simulink model "mpc_v0_1"  (R2020b)
settings: Solver=ode4  StartTime=0.0  StopTime=t_sim  FixedStep=T  RelTol=1e-3
values from neighbouring files (symbols this model uses):
  ref = [18; 9; 0; 0]    [main_01.m]
  T = 0.01    [main_01.m]
  x0 = [1; 1; 0; 0]    [main_01.m]
undefined symbols (not defined in the file or in its folder): map, mpc, mpc_param
settings Model: SimulationMode=accelerator  Creator=vince  LastModifiedBy=vince
settings DataIOCC: ReturnWorkspaceOutputs=off

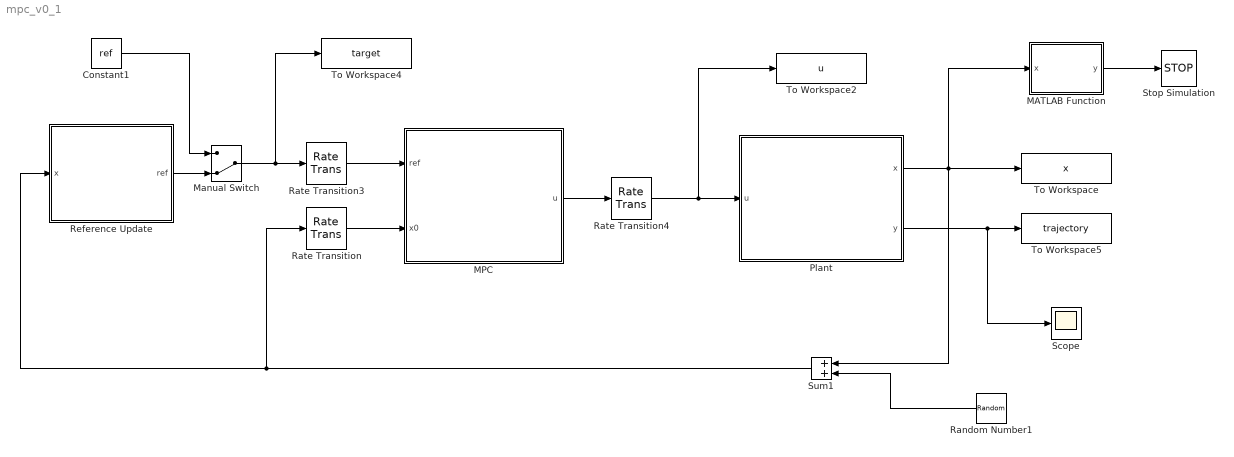
== system mpc_v0_1 ==
  Constant1 : Constant  Value=ref  SampleTime=-1
  MATLAB Function : MATLAB Function  TreatAsAtomicUnit=on
  MPC : Subsystem
  Manual Switch : ManualSwitch  CurrentSetting=0
  Plant : Subsystem
  Random Number1 : RandomNumber  Variance=0
  Rate Transition : RateTransition  OutPortSampleTime=mpc.Ts
  Rate Transition3 : RateTransition  OutPortSampleTime=mpc.Ts
  Rate Transition4 : RateTransition  OutPortSampleTime=T
  Reference Update : Subsystem
  Scope : Scope
  Stop Simulation : Stop
  Sum1 : Sum
  To Workspace : ToWorkspace  VariableName=x  SaveFormat=Timeseries  SampleTime=-1
  To Workspace2 : ToWorkspace  VariableName=u  SaveFormat=Timeseries  SampleTime=-1
  To Workspace4 : ToWorkspace  VariableName=target  SaveFormat=Timeseries  SampleTime=-1
  To Workspace5 : ToWorkspace  VariableName=trajectory  SaveFormat=Timeseries  SampleTime=-1
  wires:
  Rate Transition4/1 -> To Workspace2/1, Plant/1(u)
  MPC/1(u) -> Rate Transition4/1
  Rate Transition3/1 -> MPC/1(ref)
  Rate Transition/1 -> MPC/2(x0)
  Plant/2(y) -> Scope/1, To Workspace5/1
  Reference Update/1(ref) -> Manual Switch/2
  Constant1/1 -> Manual Switch/1
  Manual Switch/1 -> To Workspace4/1, Rate Transition3/1
  MATLAB Function/1(y) -> Stop Simulation/1
  Plant/1(x) -> Sum1/1, MATLAB Function/1(x), To Workspace/1
  Random Number1/1 -> Sum1/2
  Sum1/1 -> Rate Transition/1, Reference Update/1(x)

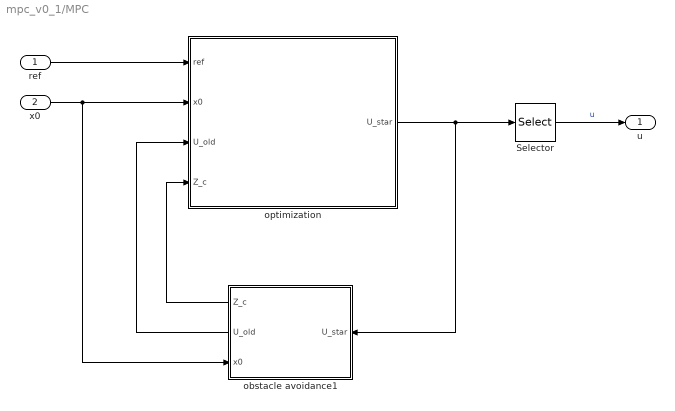
== system mpc_v0_1/MPC ==
  ref : Inport
  x0 : Inport  Port=2
  Selector : Selector  InputPortWidth=mpc.q*mpc.Nc  IndexOptions=Index vector (dialog)  Indices=1:mpc.q  OutputSizes=1
  obstacle avoidance1 : Subsystem
      settings: PortSchema="{\"entries\":[{\"content\":{\"sides\":[{\"content\":{\"connectorIds\":[\"Out1\",\"Out2\",\"In1\"]},\"type\":\"ConnectorPlacement.EquallySpacedRectSide\",\"uuid\":\"6e6bb291-76b9-457f-8d04-015292ad1700\"},{\"content\":{\"connectorIds\":[\"In2\"],\"side\":\"RIGHT\"},\"type\":\"ConnectorPlacement.EquallySpacedRectSide\",\"uuid\":\"1fce423a-e385-4f15-9cbd-eabef89b0aaa\"},{\"content\":{\"connectorIds\":[],\"side\":\"TOP\"},\"type\":\"ConnectorPlacement.EquallySpacedRectSide\",\"uuid\":\"fdf64715-349b-4f23-8b41-9be7dc47d341\"},{\"content\":{\"connectorIds\":[],\"side\":\"HIDDEN\"},\"type\":\"ConnectorPlacement.EquallySpacedRectSide\",\"uuid\":\"ad220cca-5aec-45e2-9094-855ca00bdb40\"}]},\"type\":\"ConnectorPlacement.EquallySpacedConnector\",\"uuid\":\"3c5e2d21-75ff-4523-ba4d-4cc947bcae8c\"}],\"packageUris\":[\"http://schema.mathworks.com/mf0/Connector/R2020b\"],\"version\":\"1.0\"}"
  optimization : MATLAB Function  TreatAsAtomicUnit=on
  u : Outport
  wires:
  ref/1 -> optimization/1(ref)
  x0/1 -> obstacle avoidance1/1(x0), optimization/2(x0)
  Selector/1 -> u/1  "u"
  obstacle avoidance1/1(Z_c) -> optimization/4(Z_c)
  optimization/1(U_star) -> obstacle avoidance1/2(U_star), Selector/1
  obstacle avoidance1/2(U_old) -> optimization/3(U_old)

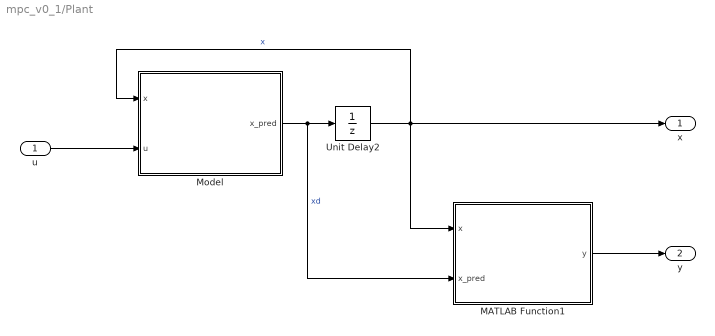
== system mpc_v0_1/Plant ==
  u : Inport
  MATLAB Function1 : MATLAB Function  TreatAsAtomicUnit=on
  Model : MATLAB Function  TreatAsAtomicUnit=on
  Unit Delay2 : UnitDelay  InitialCondition=x0  SampleTime=T  HasFrameUpgradeWarning=on
  x : Outport
  y : Outport  Port=2
  wires:
  u/1 -> Model/2(u)
  Unit Delay2/1 -> MATLAB Function1/1(x), Model/1(x), x/1  "x"
  MATLAB Function1/1(y) -> y/1
  Model/1(x_pred) -> MATLAB Function1/2(x_pred), Unit Delay2/1  "xd"

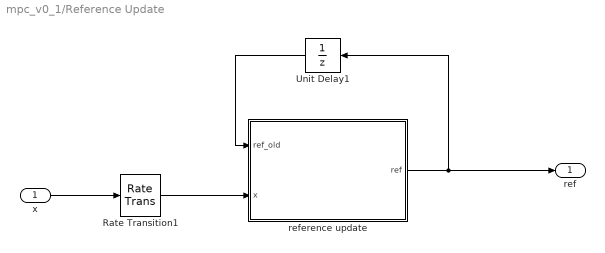
== system mpc_v0_1/Reference Update ==
  x : Inport
  Rate Transition1 : RateTransition  OutPortSampleTime=T
  Unit Delay1 : UnitDelay  InitialCondition=zeros(mpc_param.p,1)  SampleTime=T  HasFrameUpgradeWarning=on
  reference update : MATLAB Function  TreatAsAtomicUnit=on
  ref : Outport
  wires:
  Unit Delay1/1 -> reference update/1(ref_old)
  x/1 -> Rate Transition1/1
  reference update/1(ref) -> Unit Delay1/1, ref/1
  Rate Transition1/1 -> reference update/2(x)

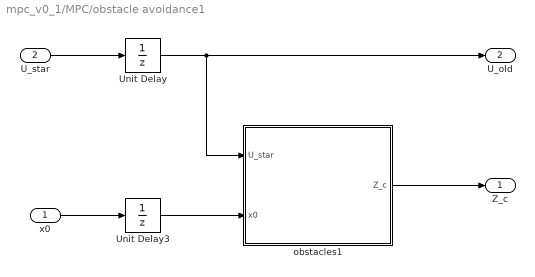
== system mpc_v0_1/MPC/obstacle avoidance1 ==
  x0 : Inport
  U_star : Inport  Port=2
  Unit Delay : UnitDelay  InitialCondition=zeros(mpc.q*mpc.Nc, 1)  SampleTime=mpc.Ts  HasFrameUpgradeWarning=on
  Unit Delay3 : UnitDelay  InitialCondition=x0  SampleTime=mpc.Ts  HasFrameUpgradeWarning=on
  obstacles1 : MATLAB Function  TreatAsAtomicUnit=on
  Z_c : Outport
  U_old : Outport  Port=2
  wires:
  obstacles1/1(Z_c) -> Z_c/1
  U_star/1 -> Unit Delay/1
  Unit Delay3/1 -> obstacles1/2(x0)
  x0/1 -> Unit Delay3/1
  Unit Delay/1 -> obstacles1/1(U_star), U_old/1

== matlab function mpc_v0_1/MPC/obstacle avoidance1/obstacles1 ==
  data: U_star input; x0 input; Z_c output; mpc parameter; map parameter
function Z_c = obstacles(U_star, x0, mpc, map)


%% Initialization
x_c = NaN*ones(mpc.Np,2);
y_c = NaN*ones(mpc.Np,2);
z_c = zeros(mpc.p*mpc.Np, 2);



%% Predicted output
X_p = mpc.A_bar*x0 + mpc.B_bar*U_star;
X = X_p(1:4:end);
Y = X_p(2:4:end);



%% Update constraints

for j = 1:mpc.Np
    %% X_c
    k = 1;
    
    for i = 1:length(map.Sx)
        if (abs(X(j)-map.Sx(i,1))>map.r_act)
            continue;
        end
        if (map.Sx(i,2)<=Y(j) && Y(j)<=map.Sx(i,3))
            x_c(j,k) = map.Sx(i,1);
            k = k+1;
        end
        if k>2
            break;
        end
    end
    

    if (isnan(x_c(j,1)) && isnan(x_c(j,2)))
        x_c(j,:) = [-Inf +Inf];
    elseif (isnan(x_c(j,2)) && X(j)>x_c(j,1))
        x_c(j,1) = x_c(j,1);
        x_c(j,2) = +Inf;
    elseif (isnan(x_c(j,2)) && X(j)<x_c(j,1))
        x_c(j,2) = x_c(j,1);
        x_c(j,1) = -Inf;
    end
    
    
    
    %% Y_c
    k = 1;

    for i=1:length(map.Sy)
        if (abs(Y(j)-map.Sy(i,1))>map.r_act)
            continue;
        end
        
        if (map.Sy(i,2)<=X(j) && X(j)<=map.Sy(i,3))
            y_c(j,k) = map.Sy(i,1);
            k = k+1;
        end
          
        if k>2
            break;
        end
    end
    
    
    if (isnan(y_c(j,1)) && isnan(y_c(j,2)))
        y_c(j,:) = [-Inf +Inf];
    elseif (isnan(y_c(j,2)) && Y(j)>y_c(j,1))
        y_c(j,1) = y_c(j,1);
        y_c(j,2) = +Inf;
    elseif (isnan(y_c(j,2)) && Y(j)<y_c(j,1))
        y_c(j,2) = y_c(j,1);
        y_c(j,1) = -Inf;
    end
    
    
    %% 
    z_c(2*j-1:2*j,:) = [x_c(j,1)+map.r_safe x_c(j,2)-map.r_safe; 
                        y_c(j,1)+map.r_safe y_c(j,2)-map.r_safe];


end


% X_min = x_c(1,1);
% X_max = x_c(1,2);
% Y_min = y_c(1,1);
% Y_max = y_c(1,2);

Z_c = z_c;

== matlab function mpc_v0_1/MPC/optimization ==
  data: ref input; U_star output; x0 input; U_old input; Z_c input; mpc parameter
function U_star   = mpc_optimization(ref, x0, U_old, Z_c, mpc)
%% Documentation
%{
    IN: ref, x, U_old
    OUT: U*
%}


%% Reference
REF = repmat(ref, mpc.Np, 1);



%% Constraints
X_min = mpc.X_c(:,1);
X_max = mpc.X_c(:,2);
% for i=1:mpc.Np
%     X_min((mpc.n*i)-3:(mpc.n*i)-2, 1) = Z_c((2*i)-1:2*i, 1);
%     X_max((mpc.n*i)-3:(mpc.n*i)-2, 1) = Z_c((2*i)-1:2*i, 2);
% end
U_min = mpc.U_c(:,1);
U_max = mpc.U_c(:,2);
dU_min = mpc.dU_c(:,1);
dU_max = mpc.dU_c(:,2);

A_ineq = [-mpc.B_bar; 
          mpc.B_bar;
          -eye(mpc.q*mpc.Nc); 
          eye(mpc.q*mpc.Nc); 
          -eye(mpc.q*mpc.Nc); 
          eye(mpc.q*mpc.Nc)];
b_ineq = [-X_min+mpc.A_bar*x0; 
          X_max-mpc.A_bar*x0;
          -U_min; 
          U_max;
          -dU_min-U_old; 
          dU_max+U_old];



%% Objective function
H = mpc.R_bar + mpc.D_bar'*mpc.Q_bar*mpc.D_bar;
H = (H+H')/2;
f = (mpc.C_bar*x0-REF)'*mpc.Q_bar*(mpc.D_bar);



%% Optimization: J(u(k)) = U(k)'*H*U(k) + f'*U(k)
coder.extrinsic('quadprog');
% options = optimoptions('quadprog', 'Algorithm', 'active-set', 'Display', 'iter');

U_star = zeros(mpc.q*mpc.Nc, 1);
U_star = quadprog(H, f, A_ineq, b_ineq, [], [], [], [], []);

== matlab function mpc_v0_1/Plant/Model ==
  data: x input; u input; x_pred output; T parameter
function x_pred = mpc_pred_disc(x, u, T)


A = [0 0 1 0; 0 0 0 1; 0 0 0 0; 0 0 0 0];
B = [0 0; 0 0; 1 0; 0 1];
C = eye(4);
D = zeros(size(C,1), size(B,2));

% Discretization
Ad = eye(size(A))+A*T;
Bd = B*T;
Cd = C;
Dd = D;

x_pred = Ad*x + Bd*u;

== matlab function mpc_v0_1/MATLAB Function ==
  data: x input; y output; wp parameter
function y = stop_sim(x, wp)

y = 0;
target = wp.points(:,end);

if (abs(x(1)-target(1))<=wp.tol && abs(x(2)-target(2))<=wp.tol)
    y = 1;
end

== matlab function mpc_v0_1/Reference Update/reference update ==
  data: ref_old input; x input; ref output; wp parameter
function ref  = ref_update(ref_old, x, wp)


for i=1:length(wp.points)-1
    
    ref = ref_old;
    
    if (ref_old==zeros(size(ref_old)))
        % Set first waypoint
        ref = [wp.points(1:2,1); x(3:4)];
        break;
    elseif (ref_old(1:2) == wp.points(:,end))
        % Update waypoint
        ref = [ref_old(1:2); x(3:4)];
        break;
    elseif(abs(x(1)-wp.points(1,i))<wp.tol && abs(x(2)-wp.points(2,i))<wp.tol)
        % No updating
        ref = [wp.points(1:2,i+1); x(3:4)];
        break;
    end
    
end

== matlab function mpc_v0_1/Plant/MATLAB Function1 ==
  data: x input; y output; x_pred input
function y = point_model_trasformation(x, x_pred)

theta = atan2((x_pred(2)-x(2)), (x_pred(1)-x(1)));
theta = theta*180/pi;
v = sqrt(x(3)^2+x(4)^2);
y = [x(1); x(2); theta; v];
